simulink model "robotController2"  (R2021b)
settings: Solver=VariableStepAuto  StartTime=0.0  StopTime=10.0  RelTol=1e-3
undefined symbols (not defined in the file): goalCheckDistance, initTheta, initX, initY, lidarScnAngls, map, prmConnectionDistance, prmMaxWaypoints, prmNumNodes, scanAngles
libraries: simulink x4, robotalgslib x2
settings Model: Creator=yekin  LastModifiedBy=yekin

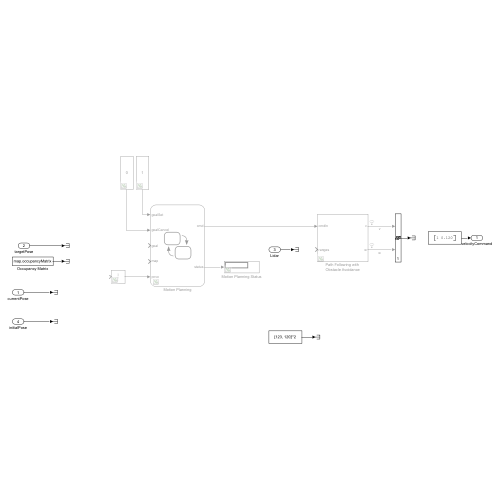
[thumbnail: Simulink's stored preview of the top-level diagram]
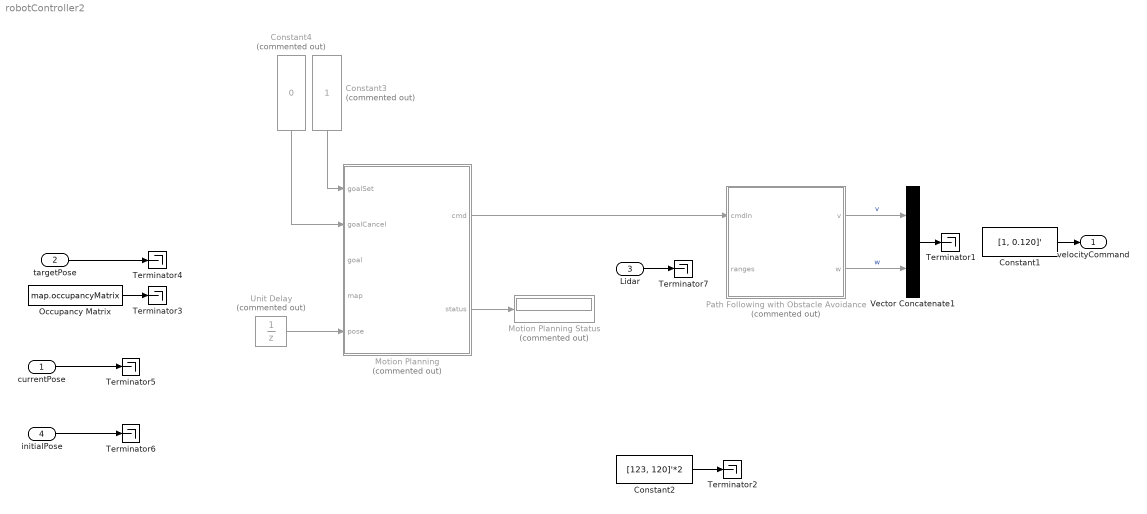
== system robotController2 ==
  currentPose : Inport  PortDimensions=3
  targetPose : Inport  Port=2  PortDimensions=3
  Lidar : Inport  Port=3  PortDimensions=length(lidarScnAngls)
  initialPose : Inport  Port=4  PortDimensions=3
  Constant1 : Constant  Value=[1, 0.120]'
  Constant2 : Constant  Value=[123, 120]'*2
  Constant3 : Constant  Commented=on
  Constant4 : Constant  Commented=on  Value=0
  Motion Planning : Stateflow chart  Commented=on  TreatAsAtomicUnit=on
  Motion Planning Status : Display  Commented=on
  Occupancy Matrix : Constant  Value=map.occupancyMatrix
  Path Following with Obstacle Avoidance : Subsystem  Commented=on
  Terminator{1..7} (7 alike) : Terminator
  Unit Delay : UnitDelay  Commented=on  InitialCondition=[initX;initY;initTheta]  SampleTime=-1  HasFrameUpgradeWarning=on
  Vector Concatenate1 : Concatenate  Mode=Multidimensional array
  velocityCommand : Outport
  wires:
  Constant2/1 -> Terminator2/1
  Path Following with Obstacle Avoidance/2(w) -> Vector Concatenate1/2  "w"
  Motion Planning/1(cmd) -> Path Following with Obstacle Avoidance/1(cmdIn)
  Constant4/1 -> Motion Planning/2(goalCancel)
  Path Following with Obstacle Avoidance/1(v) -> Vector Concatenate1/1  "v"
  Motion Planning/2(status) -> Motion Planning Status/1
  Constant3/1 -> Motion Planning/1(goalSet)
  Unit Delay/1 -> Motion Planning/5(pose)
  Vector Concatenate1/1 -> Terminator1/1
  Constant1/1 -> velocityCommand/1
  Occupancy Matrix/1 -> Terminator3/1
  targetPose/1 -> Terminator4/1
  currentPose/1 -> Terminator5/1
  Lidar/1 -> Terminator7/1
  initialPose/1 -> Terminator6/1

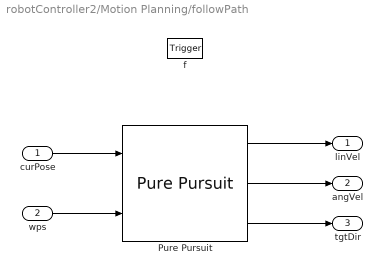
== system robotController2/Motion Planning/followPath ==
  curPose : Inport  OutDataTypeStr=double  PortDimensions=3
  wps : Inport  Port=2  OutDataTypeStr=double  PortDimensions=[prmMaxWaypoints 2]
      settings: VarSizeSig=Yes
  f : TriggerPort  TriggerType=function-call  VariantControl=(inherit)
      settings: CopyFcn=Stateflow.SLINSF.SimulinkMan.removeBlockPreDeleteFcn  PreDeleteFcn=Stateflow.SLINSF.SimulinkMan.unsafePredeleteFcn
  Pure Pursuit : robotalgslib/Pure Pursuit  DesiredLinearVelocity=followerLinSpeed  MaxAngularVelocity=followerMaxAngSpeed  LookaheadDistance=followerLookaheadDistance  TargetDirPort=on  SimulateUsing=Interpreted execution
  linVel : Outport  PortDimensions=1
  angVel : Outport  Port=2  PortDimensions=1
  tgtDir : Outport  Port=3  PortDimensions=1
  wires:
  curPose/1 -> Pure Pursuit/1
  wps/1 -> Pure Pursuit/2
  Pure Pursuit/2 -> angVel/1
  Pure Pursuit/3 -> tgtDir/1
  Pure Pursuit/1 -> linVel/1

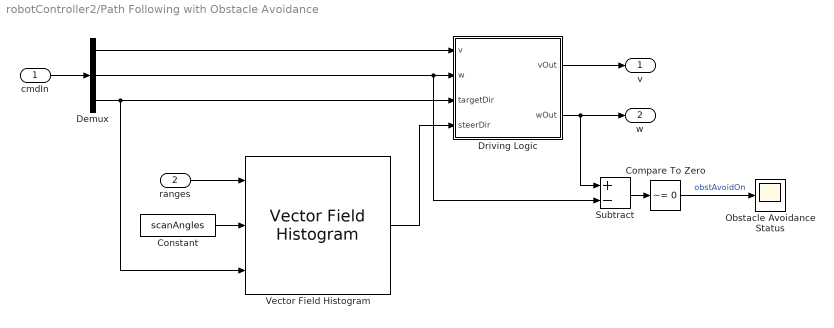
== system robotController2/Path Following with Obstacle Avoidance ==
  cmdIn : Inport
  ranges : Inport  Port=2
  Compare To Zero : simulink/Logic and Bit Operations/Compare To Zero  relop=~=  OutDataTypeStr=boolean
  Constant : Constant  Value=scanAngles
  Demux : Demux  Outputs=3
  Driving Logic : Subsystem
  Obstacle Avoidance Status : Scope
  Subtract : Sum  Inputs=+-
  Vector Field Histogram : robotalgslib/Vector Field Histogram  NumAngularSectors=10  DistanceLimits=[ 0.05, 3 ]  HistogramThresholds=[ 1, 2 ]  RobotRadius=0.25  SafetyDistance=0.5  MinTurningRadius=0.2  SimulateUsing=Interpreted execution  TargetDirectionWeight=5  CurrentDirectionWeight=2  PreviousDirectionWeight=2
      settings: SourceProductBaseCode=NV,RO
  v : Outport  VectorParamsAs1DForOutWhenUnconnected=off
  w : Outport  Port=2  VectorParamsAs1DForOutWhenUnconnected=off
  wires:
  cmdIn/1 -> Demux/1
  Demux/3 -> Vector Field Histogram/3, Driving Logic/3(targetDir)
  Demux/1 -> Driving Logic/1(v)
  Constant/1 -> Vector Field Histogram/2
  Vector Field Histogram/1 -> Driving Logic/4(steerDir)
  ranges/1 -> Vector Field Histogram/1
  Driving Logic/1(vOut) -> v/1
  Demux/2 -> Subtract/2, Driving Logic/2(w)
  Driving Logic/2(wOut) -> w/1, Subtract/1
  Compare To Zero/1 -> Obstacle Avoidance Status/1  "obstAvoidOn"
  Subtract/1 -> Compare To Zero/1

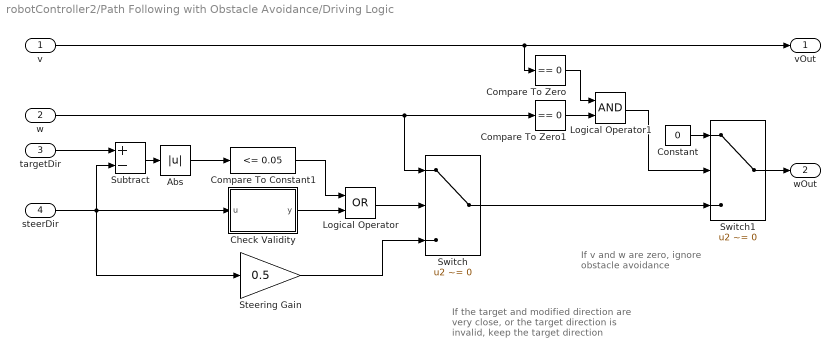
== system robotController2/Path Following with Obstacle Avoidance/Driving Logic ==
  note: If v and w are zero, ignore obstacle avoidance
  note: If the target and modified direction are very close, or the target direction is invalid, keep the target direction
  v : Inport
  w : Inport  Port=2
  targetDir : Inport  Port=3
  steerDir : Inport  Port=4
  Abs : Abs
  Check Validity : MATLAB Function  TreatAsAtomicUnit=on
  Compare To Constant1 : simulink/Logic and Bit Operations/Compare To Constant  relop=<=  const=0.05  OutDataTypeStr=boolean
  Compare To Zero : simulink/Logic and Bit Operations/Compare To Zero  relop===  OutDataTypeStr=boolean
  Compare To Zero1 : simulink/Logic and Bit Operations/Compare To Zero  relop===  OutDataTypeStr=boolean
  Constant : Constant  Value=0
  Logical Operator : Logic  Operator=OR  AllPortsSameDT=off  OutDataTypeStr=boolean
  Logical Operator1 : Logic  AllPortsSameDT=off  OutDataTypeStr=boolean
  Steering Gain : Gain  Gain=0.5
  Subtract : Sum  Inputs=+-
  Switch : Switch  Criteria=u2 ~= 0
  Switch1 : Switch  Criteria=u2 ~= 0
  vOut : Outport  VectorParamsAs1DForOutWhenUnconnected=off
  wOut : Outport  Port=2  VectorParamsAs1DForOutWhenUnconnected=off
  wires:
  steerDir/1 -> Steering Gain/1, Check Validity/1(u), Subtract/2
  Check Validity/1(y) -> Logical Operator/2
  targetDir/1 -> Subtract/1
  Subtract/1 -> Abs/1
  Abs/1 -> Compare To Constant1/1
  Compare To Constant1/1 -> Logical Operator/1
  Logical Operator/1 -> Switch/2
  w/1 -> Switch/1, Compare To Zero1/1
  Switch/1 -> Switch1/3
  Steering Gain/1 -> Switch/3
  Switch1/1 -> wOut/1
  v/1 -> Compare To Zero/1, vOut/1
  Compare To Zero1/1 -> Logical Operator1/2
  Compare To Zero/1 -> Logical Operator1/1
  Logical Operator1/1 -> Switch1/2
  Constant/1 -> Switch1/1

== matlab function robotController2/Path Following with Obstacle Avoidance/Driving Logic/Check Validity ==
  data: u input; y output
function y = checkValid(u)

y = isnan(u);

== stateflow chart robotController2/Motion Planning ==
  settings: updateMethod=DISCRETE  sampleTime=sampleTime
  state ExecuteMotionPlan
    (default) -> (junction 45) : {pathFound = false;}
    ExecuteMotionPlan -> (junction 45) [order 1]
    (junction 45) -> (junction 48) [order 1] : [pathFound]
    (junction 45) -> (junction 52) [order 2] : % Plan a path
        | {
        | [waypoints,pathFound] = ...
        | computePath(goal,pose,map);
        | }
    (junction 48) -> (junction 50) : % If a path exists, follow it
        | {
        | [v,w,d] = followPath(pose,waypoints);
        | cmd = [v;w;d];
        | status = MotionPlanning.FOLLOWING;
        | }
    (junction 50) -> (junction 52)
  state Standby
    en:
    cmd = [0;0;0];
  state done = isGoalReached [function]
    (default) -> (junction 30) : {
        | dist = sqrt((goal(1)-pose(1))^2 + (goal(2)-pose(2))^2);
        | done = (dist <= goalCheckDistance);
        | }
  state [linVel,angVel,tgtDir]  = followPath(curPose,wps) [function]
  (default) -> Standby
  Standby -> ExecuteMotionPlan : [hasChangedTo(goalSet,true)]
  ExecuteMotionPlan -> Standby [order 1] : % Goal is successfully reached
      | [isGoalReached]
      | {status = MotionPlanning.SUCCESS;}
  ExecuteMotionPlan -> Standby [order 2] : % User cancels motion planning
      | [hasChangedTo(goalCancel,true)]
      | {status = MotionPlanning.CANCELLED;}
  ExecuteMotionPlan -> Standby [order 3] : % Exit if path planning fails multiple times
      | [after(10,tick) && ~pathFound]
      | {status = MotionPlanning.FAILED;}
  data: done function_output; wps function_output; tgtPose function_input; curPose function_input; occMat function_input; found function_output; curPose function_input double size=3; wps function_input double size=[prmMaxWaypoints 2]; linVel function_output size=1; angVel function_output size=1; tgtDir function_output size=1; cmd output; goalSet input; goalCancel input; goal input; map input; pose input; waypoints local size=[prmMaxWaypoints 2]; status output =MotionPlanning.UNASSIGNED; pathFound local; prmConnectionDistance parameter; prmNumNodes parameter; goalCheckDistance parameter; d local; v local; w local
  function [wps,found] = computePath(tgtPose,curPose,occMat):
    | function [wps,found] = computePath(tgtPose,curPose,occMat)
    | 
    | % Initialize path planner on initialization
    | coder.extrinsic('showPath')
    | persistent planner firstTime
    | if isempty(planner)
    |     occMap = occupancyMap(occMat,2);
    |     planner = mobileRobotPRM(occMap);
    |     % inflate(occMap,0.2); % No inflation in this example, obstacle avoidance handles it
    |     planner.ConnectionDistance = prmConnectionDistance;
    |     planner.NumNodes = prmNumNodes;
    |     firstTime = true;
    | end
    | 
    | % Validate the input
    | found = false;
    | if (tgtPose(1) >= planner.Map.XWorldLimits(1)) && (tgtPose(1) <= planner.Map.XWorldLimits(2)) && ...
    |         (tgtPose(2) >= planner.Map.YWorldLimits(1)) && (tgtPose(2) <= planner.Map.YWorldLimits(2)) && ...
    |         (~checkOccupancy(planner.Map,[tgtPose(1) tgtPose(2)]))
    |     
    |     % If this is not the first time using the PRM, but the previous path
    |     % failed, then increase the number of nodes in the PRM and try again.
    |     if ~firstTime
    |         planner.NumNodes = planner.NumNodes + prmNumNodes;
    |     end
    |     
    |     % Find a path given start and end positions
    |     wps = findpath(planner,[curPose(1) curPose(2)],[tgtPose(1) tgtPose(2)]);
    |     
    |     % Path is successfully found if the output of "findpath" is non-empty
    |     if ~isempty(wps)
    |         found = true;
    |         planner.NumNodes = prmNumNodes;
    |         showPath(wps);
    |     else
    |         firstTime = false;
    |     end
    | else
    |     wps = [];  
    | end
